simulink model "fuckingAround"  (R2019b)
settings: Solver=ode8  StartTime=0.0  StopTime=2.5  FixedStep=0.05  RelTol=1e-3
undefined symbols (not defined in the file or in its folder): aero, fa, fde, fdelL, fh, fm, idxa, idxde, idxdelL, idxh, idxm
libraries: aerolibconvert2 x3, aerolibasang x3, aerolibadyn x2, shared6dof x1
settings Model: SnapshotInterval=1  Creator=fberbari  LastModifiedBy=Antho
settings DataIOCC: ReturnWorkspaceOutputs=off
settings DebuggingCC: ArithmeticOperatorsInVariantConditions=warning
settings SFSimCC: DefaultCustomCodeFunctionArrayLayout=Row-major  CustomCodeUndefinedFunction=UseInterfaceOnly
settings RTWCC: GenCodeOnly=on  PackageGeneratedCodeAndArtifacts=on  PackageName=GeneratedCCode.zip  TargetLang=C++
settings GRTTargetCC: TargetLangStandard=C++03 (ISO)  MatFileLogging=off  MultiInstanceERTCode=on  CodeInterfacePackaging=C++ class

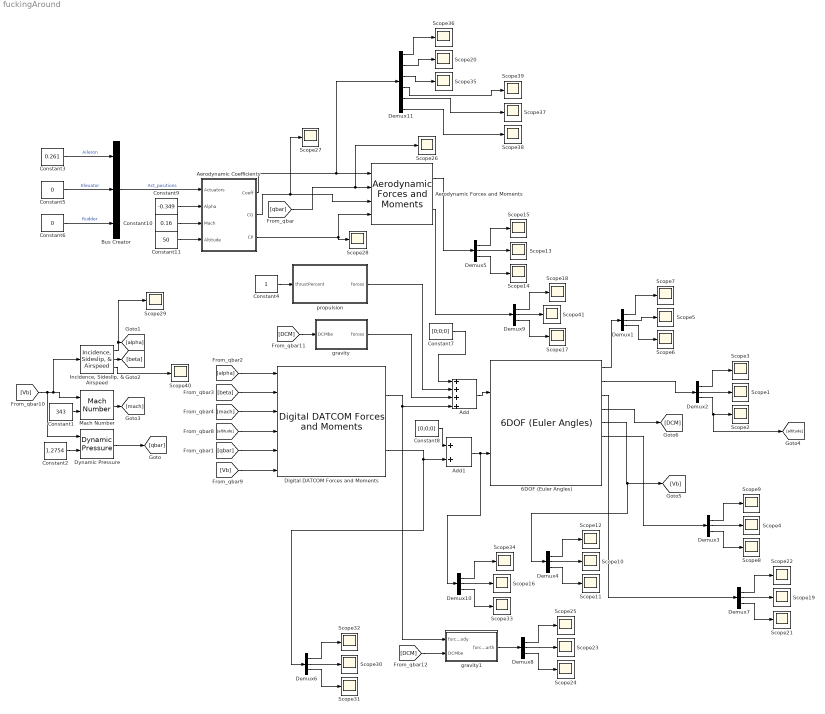
== system fuckingAround ==
  6DOF (Euler Angles) : shared6dof/6DOF (Euler Angles)  units=Metric (MKS)  mtype=Fixed  rep=Euler Angles  xme_0=[0 0 150]  Vm_0=[60 0 0]  eul_0=[0 0 0]  pm_0=[0 0 0]  mass_0=800  mass_e=0.5  mass_f=2.0  inertia=[1541 0 0; 0 1898 0; 0 0 3199]  inertia_e=eye(3)  inertia_f=2*eye(3)  k_quat=1.0  vre_flag=on  abi_flag=on  aMode=0  xme_statename=''  Vm_statename=''  eul_statename=''  quat_statename=''  pm_statename=''  mass_statename=''
      settings: SourceProductBaseCode=AE
  Add : Sum  Inputs=++++
  Add1 : Sum
  Aerodynamic Coefficients : Subsystem
  "Aerodynamic Forces and Moments " : aerolibadyn/Aerodynamic Forces and Moments   inputAxes=Body  outputForceAxes=Body  outputMomentAxes=Body  S=aero{1}.sref  b=aero{1}.blref  cbar=aero{1}.cbar
      settings: SourceProductName=Aerospace Blockset
  Bus Creator : BusCreator  Inputs=3
  Constant1 : Constant  Value=343
  Constant10 : Constant  Value=0.16
  Constant11 : Constant  Value=50
  Constant2 : Constant  Value=1.2754
  Constant3 : Constant  Value=0.261
  Constant4 : Constant
  Constant5 : Constant  Value=0
  Constant6 : Constant  Value=0
  Constant7 : Constant  Value=[0;0;0]
  Constant8 : Constant  Value=[0;0;0]
  Constant9 : Constant  Value=-0.349
  Demux{1..10} (10 alike) : Demux  Outputs=3
  Demux11 : Demux  Outputs=6
  Digital DATCOM Forces and Moments : aerolibadyn/Digital DATCOM Forces and Moments  units=Metric (MKS)  dcase=aero{1}  fmode=Body  buildno=0  imethod=Linear  emethod=Linear  rmethod=Linear Extrapolation  action=Error
      settings: SourceProductName=Aerospace Blockset  SourceProductBaseCode=AE
  Dynamic Pressure : aerolibasang/Dynamic Pressure
  "Incidence, Sideslip, & Airspeed" : aerolibasang/Incidence, Sideslip, & Airspeed
      settings: SourceProductName=Aerospace Blockset
  Mach Number : aerolibasang/Mach Number
      settings: SourceProductName=Aerospace Blockset  SourceProductBaseCode=AE
  Scope{1..41} (41 alike) : Scope
  gravity : MATLAB Function  TreatAsAtomicUnit=on
  gravity1 : MATLAB Function  TreatAsAtomicUnit=on
  propulsion : MATLAB Function  TreatAsAtomicUnit=on
  wires:
  Constant2/1 -> Dynamic Pressure/2
  Constant1/1 -> Mach Number/2
  Demux1/2 -> Scope5/1
  Demux1/3 -> Scope6/1
  Demux1/1 -> Scope7/1
  6DOF (Euler Angles)/1 -> Demux1/1
  Demux2/1 -> Scope3/1
  Demux2/2 -> Scope1/1
  6DOF (Euler Angles)/2 -> Demux2/1
  Demux2/3 -> [altitude], Scope2/1
  Demux3/1 -> Scope9/1
  Demux3/3 -> Scope8/1
  Demux3/2 -> Scope4/1
  6DOF (Euler Angles)/6 -> Demux3/1
  Demux4/3 -> Scope11/1
  Demux4/2 -> Scope10/1
  Demux4/1 -> Scope12/1
  Demux5/1 -> Scope15/1
  Demux5/3 -> Scope14/1
  Demux5/2 -> Scope13/1
  Demux7/2 -> Scope19/1
  Demux7/1 -> Scope22/1
  Demux7/3 -> Scope21/1
  6DOF (Euler Angles)/3 -> Demux7/1
  Constant4/1 -> propulsion/1(thrustPercent)
  Demux8/1 -> Scope25/1
  Demux8/3 -> Scope24/1
  Demux8/2 -> Scope23/1
  Demux6/2 -> Scope30/1
  Demux6/3 -> Scope31/1
  Demux6/1 -> Scope32/1
  Digital DATCOM Forces and Moments/2 -> Demux6/1, Add1/2
  Aerodynamic Coefficients/3(CP) -> "Aerodynamic Forces and Moments "/4, Scope28/1
  Aerodynamic Coefficients/2(CG) -> "Aerodynamic Forces and Moments "/3, Scope27/1
  [qbar] -> Scope26/1, "Aerodynamic Forces and Moments "/2
  [qbar] -> Digital DATCOM Forces and Moments/5
  Dynamic Pressure/1 -> [qbar]
  "Incidence, Sideslip, & Airspeed"/1 -> Scope29/1, [alpha]
  "Incidence, Sideslip, & Airspeed"/2 -> [beta]
  [alpha] -> Digital DATCOM Forces and Moments/1
  [beta] -> Digital DATCOM Forces and Moments/2
  Mach Number/1 -> [mach]
  [mach] -> Digital DATCOM Forces and Moments/3
  Constant10/1 -> Aerodynamic Coefficients/3(Mach)
  Constant9/1 -> Aerodynamic Coefficients/2(Alpha)
  Constant11/1 -> Aerodynamic Coefficients/4(Altitude)
  [altitude] -> Digital DATCOM Forces and Moments/4
  6DOF (Euler Angles)/5 -> Demux4/1, [Vb]
  [Vb] -> Digital DATCOM Forces and Moments/6
  [Vb] -> Dynamic Pressure/1, "Incidence, Sideslip, & Airspeed"/1, Mach Number/1
  Add/1 -> 6DOF (Euler Angles)/1
  "Aerodynamic Forces and Moments "/1 -> Demux5/1
  propulsion/1(forces) -> Add/2
  Digital DATCOM Forces and Moments/1 -> gravity1/1(forcesBody), Add/4
  gravity/1(forces) -> Add/3
  6DOF (Euler Angles)/4 -> [DCM]
  [DCM] -> gravity/1(DCMbe)
  "Aerodynamic Forces and Moments "/2 -> Demux9/1
  Constant5/1 -> Bus Creator/2  "Elevator"
  Constant6/1 -> Bus Creator/3  "Rudder"
  Bus Creator/1 -> Aerodynamic Coefficients/1(Actuators)  "Act_positions"
  Constant3/1 -> Bus Creator/1  "Aileron"
  Demux9/3 -> Scope17/1
  Demux9/1 -> Scope18/1
  Demux9/2 -> Scope41/1
  Demux10/2 -> Scope16/1
  Demux10/3 -> Scope33/1
  Add1/1 -> Demux10/1, 6DOF (Euler Angles)/2
  Demux10/1 -> Scope34/1
  Demux11/2 -> Scope20/1
  Demux11/3 -> Scope35/1
  Aerodynamic Coefficients/1(Coeff) -> Demux11/1, "Aerodynamic Forces and Moments "/1
  Demux11/1 -> Scope36/1
  Demux11/4 -> Scope39/1
  Demux11/5 -> Scope37/1
  Demux11/6 -> Scope38/1
  "Incidence, Sideslip, & Airspeed"/3 -> Scope40/1
  gravity1/1(forcesEarth) -> Demux8/1
  [DCM] -> gravity1/2(DCMbe)
  Constant7/1 -> Add/1
  Constant8/1 -> Add1/1

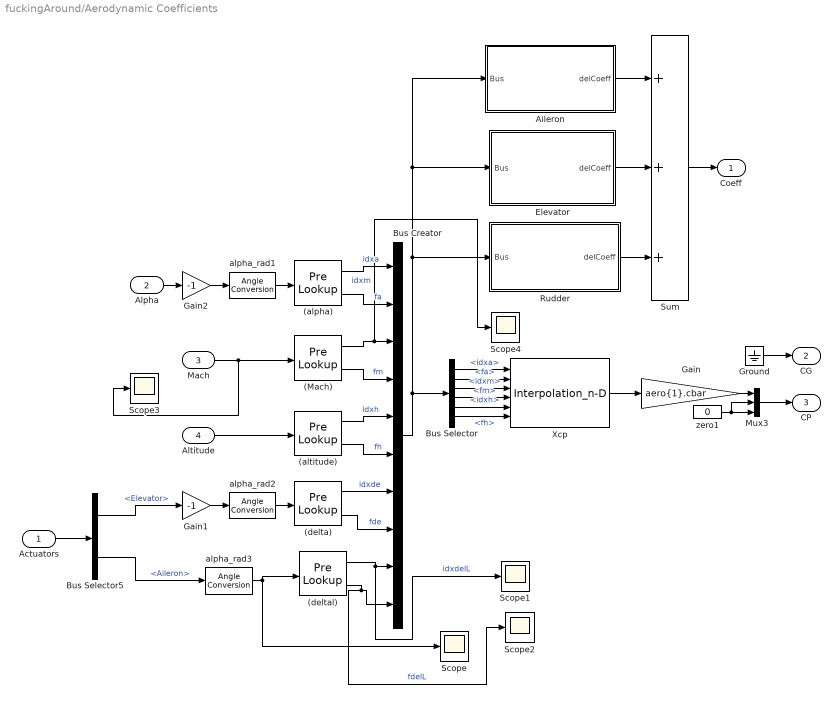
== system fuckingAround/Aerodynamic Coefficients ==
  Actuators : Inport
  Alpha : Inport  Port=2
  Mach : Inport  Port=3
  Altitude : Inport  Port=4
  (Mach) : PreLookup  BreakpointsData=aero{1}.mach  BeginIndexSearchUsingPreviousIndexResult=on  ExtrapMethod=Linear  IndexDataTypeStr=int32  FractionDataTypeStr=double
  (alpha) : PreLookup  BreakpointsData=aero{1}.alpha  BeginIndexSearchUsingPreviousIndexResult=on  ExtrapMethod=Linear  IndexDataTypeStr=int32  FractionDataTypeStr=double
  (altitude) : PreLookup  BreakpointsData=aero{1}.alt  BeginIndexSearchUsingPreviousIndexResult=on  ExtrapMethod=Linear  IndexDataTypeStr=int32  FractionDataTypeStr=double
  (delta) : PreLookup  BreakpointsData=aero{1}.delta  BeginIndexSearchUsingPreviousIndexResult=on  ExtrapMethod=Linear  IndexDataTypeStr=int32  FractionDataTypeStr=double
  (deltal) : PreLookup  BreakpointsData=aero{2}.deltal  BeginIndexSearchUsingPreviousIndexResult=on  ExtrapMethod=Linear  IndexDataTypeStr=int32  FractionDataTypeStr=double
  Aileron : Subsystem
  Bus Creator : BusCreator  Inputs=idxa,fa,idxm,fm,idxh,fh,idxde,fde,idxdelL,fdelL
  Bus Selector : BusSelector  OutputSignals=idxa,fa,idxm,fm,idxh,fh
  Bus Selector5 : BusSelector  OutputSignals=Elevator,Aileron
  Elevator : Subsystem
  Gain : Gain  Gain=aero{1}.cbar
  Gain1 : Gain  Gain=-1
  Gain2 : Gain  Gain=-1
  Ground : Ground
  Mux3 : Mux  Inputs=3
  Rudder : Subsystem
  Scope{,1..4} (5 alike) : Scope
  Sum : Sum  Inputs=3  SaturateOnIntegerOverflow=on  InputSameDT=on  OutDataTypeStr=Inherit: Same as first input
  Xcp : Interpolation_n-D  NumberOfTableDimensions=3  Table="permute(aero{1}.xcp,[1  2  3])"  OutDataTypeStr=double
      settings: InputPortMap=u0,u1,u2,u3,u4,u5
  alpha_rad1 : aerolibconvert2/Angle Conversion  IU=rad  OU=deg
  alpha_rad2 : aerolibconvert2/Angle Conversion  IU=rad  OU=deg
  alpha_rad3 : aerolibconvert2/Angle Conversion  IU=rad  OU=deg
  zero1 : Constant  Value=0
  Coeff : Outport  InitialOutput=0  VectorParamsAs1DForOutWhenUnconnected=off
  CG : Outport  Port=2  PortDimensions=3  InitialOutput=0  VectorParamsAs1DForOutWhenUnconnected=off
  CP : Outport  Port=3  PortDimensions=3  InitialOutput=0  VectorParamsAs1DForOutWhenUnconnected=off
  wires:
  Sum/1 -> Coeff/1
  Actuators/1 -> Bus Selector5/1
  Ground/1 -> CG/1
  Mux3/1 -> CP/1
  Xcp/1 -> Gain/1
  zero1/1 -> Mux3/2, Mux3/3
  Gain/1 -> Mux3/1
  (alpha)/2 -> Bus Creator/2  "fa"
  (Mach)/2 -> Bus Creator/4  "fm"
  (altitude)/2 -> Bus Creator/6  "fh"
  (altitude)/1 -> Bus Creator/5  "idxh"
  (Mach)/1 -> Scope4/1, Bus Creator/3  "idxm"
  (alpha)/1 -> Bus Creator/1  "idxa"
  Bus Selector/1 -> Xcp/1  "<idxa>"
  Bus Selector/2 -> Xcp/2  "<fa>"
  Bus Selector/3 -> Xcp/3  "<idxm>"
  Bus Selector/4 -> Xcp/4  "<fm>"
  Bus Selector/5 -> Xcp/5  "<idxh>"
  Bus Selector/6 -> Xcp/6  "<fh>"
  Bus Creator/1 -> Bus Selector/1, Elevator/1(Bus), Aileron/1(Bus), Rudder/1(Bus)
  Mach/1 -> Scope3/1, (Mach)/1
  Altitude/1 -> (altitude)/1
  alpha_rad1/1 -> (alpha)/1
  Aileron/1(delCoeff) -> Sum/1
  Elevator/1(delCoeff) -> Sum/2
  Rudder/1(delCoeff) -> Sum/3
  (delta)/1 -> Bus Creator/7  "idxde"
  (delta)/2 -> Bus Creator/8  "fde"
  alpha_rad2/1 -> (delta)/1
  Gain1/1 -> alpha_rad2/1
  Bus Selector5/1 -> Gain1/1  "<Elevator>"
  (deltal)/1 -> Scope1/1, Bus Creator/9  "idxdelL"
  (deltal)/2 -> Scope2/1, Bus Creator/10  "fdelL"
  alpha_rad3/1 -> Scope/1, (deltal)/1
  Bus Selector5/2 -> alpha_rad3/1  "<Aileron>"
  Alpha/1 -> Gain2/1
  Gain2/1 -> alpha_rad1/1

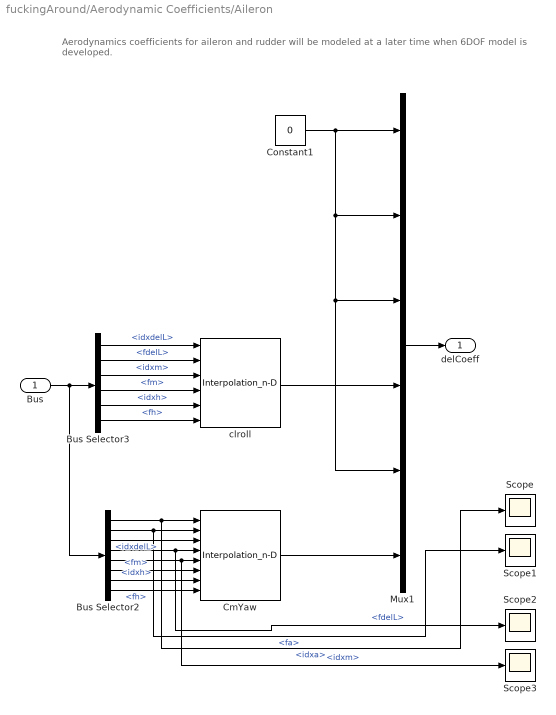
== system fuckingAround/Aerodynamic Coefficients/Aileron ==
  note: Aerodynamics coefficients for aileron and rudder will be modeled at a later time when 6DOF model is developed.
  Bus : Inport
  Bus Selector2 : BusSelector  OutputSignals=idxa,fa,idxdelL,fdelL,idxm,fm,idxh,fh
  Bus Selector3 : BusSelector  OutputSignals=idxdelL,fdelL,idxm,fm,idxh,fh
  "CmYaw " : Interpolation_n-D  NumberOfTableDimensions=4  Table=aero{2}.cn_asy  RemoveProtectionIndex=on
      settings: InputPortMap=u0,u1,u2,u3,u4,u5,u6,u7
  Constant1 : Constant  Value=0
  Mux1 : Mux  Inputs=6
  Scope{,1..3} (4 alike) : Scope
  clroll : Interpolation_n-D  NumberOfTableDimensions=3  Table="permute(aero{2}.clroll,[1  2  3])"  RemoveProtectionIndex=on
      settings: InputPortMap=u0,u1,u2,u3,u4,u5
  delCoeff : Outport  VectorParamsAs1DForOutWhenUnconnected=off
  wires:
  Mux1/1 -> delCoeff/1
  Constant1/1 -> Mux1/1, Mux1/2, Mux1/3, Mux1/5
  clroll/1 -> Mux1/4
  Bus/1 -> Bus Selector2/1, Bus Selector3/1
  Bus Selector3/1 -> clroll/1  "<idxdelL>"
  Bus Selector3/2 -> clroll/2  "<fdelL>"
  Bus Selector3/3 -> clroll/3  "<idxm>"
  Bus Selector3/4 -> clroll/4  "<fm>"
  Bus Selector3/5 -> clroll/5  "<idxh>"
  Bus Selector3/6 -> clroll/6  "<fh>"
  "CmYaw "/1 -> Mux1/6
  Bus Selector2/1 -> Scope/1, "CmYaw "/1  "<idxa>"
  Bus Selector2/2 -> Scope1/1, "CmYaw "/2  "<fa>"
  Bus Selector2/3 -> "CmYaw "/3  "<idxdelL>"
  Bus Selector2/4 -> Scope2/1, "CmYaw "/4  "<fdelL>"
  Bus Selector2/5 -> Scope3/1, "CmYaw "/5  "<idxm>"
  Bus Selector2/6 -> "CmYaw "/6  "<fm>"
  Bus Selector2/7 -> "CmYaw "/7  "<idxh>"
  Bus Selector2/8 -> "CmYaw "/8  "<fh>"

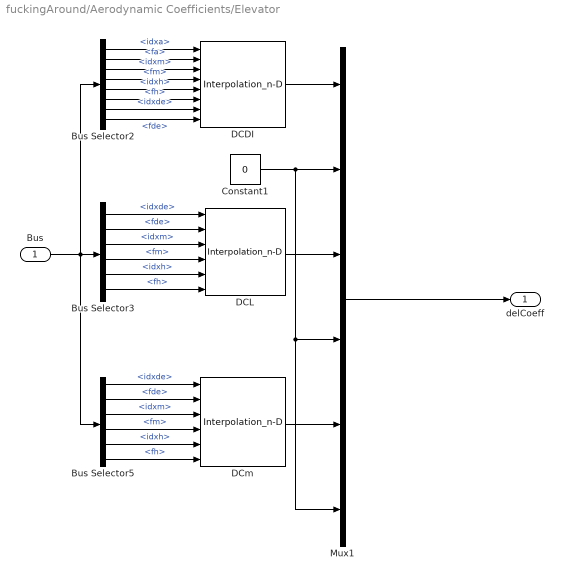
== system fuckingAround/Aerodynamic Coefficients/Elevator ==
  Bus : Inport
  Bus Selector2 : BusSelector  OutputSignals=idxa,fa,idxm,fm,idxh,fh,idxde,fde
  Bus Selector3 : BusSelector  OutputSignals=idxde,fde,idxm,fm,idxh,fh
  Bus Selector5 : BusSelector  OutputSignals=idxde,fde,idxm,fm,idxh,fh
  Constant1 : Constant  Value=0
  DCDI : Interpolation_n-D  NumberOfTableDimensions=4  Table=permute(aero{1}.dcdi_sym,[1 3 4 2 ])  RemoveProtectionIndex=on
      settings: InputPortMap=u0,u1,u2,u3,u4,u5,u6,u7
  DCL : Interpolation_n-D  NumberOfTableDimensions=3  Table="permute(aero{1}.dcl_sym,[1  2  3])"  RemoveProtectionIndex=on
      settings: InputPortMap=u0,u1,u2,u3,u4,u5
  DCm : Interpolation_n-D  NumberOfTableDimensions=3  Table="permute(aero{1}.dcm_sym,[1  2  3])"  RemoveProtectionIndex=on
      settings: InputPortMap=u0,u1,u2,u3,u4,u5
  Mux1 : Mux  Inputs=6
  delCoeff : Outport  VectorParamsAs1DForOutWhenUnconnected=off
  wires:
  Mux1/1 -> delCoeff/1
  Bus/1 -> Bus Selector2/1, Bus Selector3/1, Bus Selector5/1
  DCDI/1 -> Mux1/1
  DCL/1 -> Mux1/3
  DCm/1 -> Mux1/5
  Constant1/1 -> Mux1/2, Mux1/4, Mux1/6
  Bus Selector2/1 -> DCDI/1  "<idxa>"
  Bus Selector2/2 -> DCDI/2  "<fa>"
  Bus Selector3/1 -> DCL/1  "<idxde>"
  Bus Selector3/2 -> DCL/2  "<fde>"
  Bus Selector5/1 -> DCm/1  "<idxde>"
  Bus Selector5/2 -> DCm/2  "<fde>"
  Bus Selector2/3 -> DCDI/3  "<idxm>"
  Bus Selector2/4 -> DCDI/4  "<fm>"
  Bus Selector2/5 -> DCDI/5  "<idxh>"
  Bus Selector2/6 -> DCDI/6  "<fh>"
  Bus Selector2/7 -> DCDI/7  "<idxde>"
  Bus Selector2/8 -> DCDI/8  "<fde>"
  Bus Selector3/3 -> DCL/3  "<idxm>"
  Bus Selector3/4 -> DCL/4  "<fm>"
  Bus Selector3/5 -> DCL/5  "<idxh>"
  Bus Selector3/6 -> DCL/6  "<fh>"
  Bus Selector5/3 -> DCm/3  "<idxm>"
  Bus Selector5/4 -> DCm/4  "<fm>"
  Bus Selector5/5 -> DCm/5  "<idxh>"
  Bus Selector5/6 -> DCm/6  "<fh>"

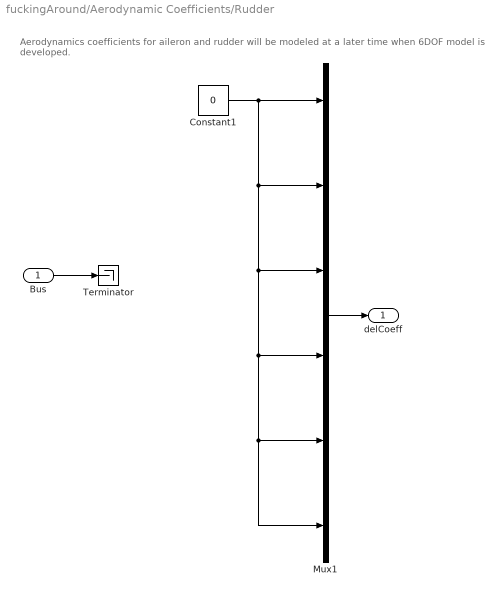
== system fuckingAround/Aerodynamic Coefficients/Rudder ==
  note: Aerodynamics coefficients for aileron and rudder will be modeled at a later time when 6DOF model is developed.
  Bus : Inport
  Constant1 : Constant  Value=0
  Mux1 : Mux  Inputs=6
  Terminator : Terminator
  delCoeff : Outport  VectorParamsAs1DForOutWhenUnconnected=off
  wires:
  Mux1/1 -> delCoeff/1
  Constant1/1 -> Mux1/6, Mux1/5, Mux1/4, Mux1/3, Mux1/2, Mux1/1
  Bus/1 -> Terminator/1

== matlab function fuckingAround/gravity ==
  data: forces output; DCMbe input
%#codegen
function forces  = fcn(DCMbe)

mass = 800;
gravityInertial = [0;0;-9.8*mass];
gravityBody = DCMbe * gravityInertial;

forces = gravityBody;

== matlab function fuckingAround/propulsion ==
  data: forces output; thrustPercent input
%#codegen
function forces  = fcn(thrustPercent)

maxThrust = 2200; %Newtons
forces = [maxThrust*thrustPercent;0;0];

== matlab function fuckingAround/gravity1 ==
  data: forcesBody input; forcesEarth output; DCMbe input
%#codegen
function forcesEarth  = fcn(forcesBody,DCMbe)



forcesEarth = DCMbe.' * forcesBody;
